simulink model "model_1"  (R2018a)
settings: Solver=VariableStepAuto  StartTime=0.0  StopTime=11  RelTol=1e-3
values from neighbouring files (symbols this model uses):
  Af = 1.8    [script.m]
  Cd = 0.25    [script.m]
  fr = 0.015    [script.m]
  g = 9.81    [script.m]
  Mv = 1310    [script.m]
  rho = 1.2    [script.m]
libraries: simulink x2
settings Model: Creator=Saurabh Suman  LastModifiedBy=Saurabh Suman

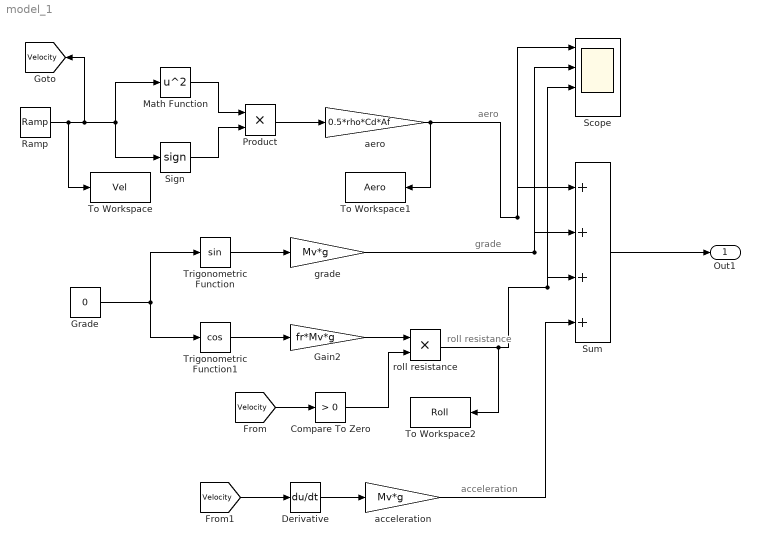
== system model_1 ==
  note: acceleration
  note: roll resistance
  note: grade
  note: aero
  Compare To Zero : simulink/Logic and Bit Operations/Compare To Zero  relop=>  OutDataTypeStr=boolean
  Derivative : Derivative
  Gain2 : Gain  Gain=fr*Mv*g
  Grade : Constant  Value=0
  Math Function : Math  Operator=square  SaturateOnIntegerOverflow=on
  Product : Product
  Ramp : simulink/Sources/Ramp  slope=10  start=1  InitialOutput=0
  Scope : Scope  NumInputPorts=4
  Sign : Signum
  Sum : Sum  Inputs=|++++
  To Workspace : ToWorkspace  VariableName=Vel  SampleTime=-1
      settings: Save2DSignal=2-D array (concatenate along first dimension)
  To Workspace1 : ToWorkspace  VariableName=Aero  SampleTime=-1
      settings: Save2DSignal=2-D array (concatenate along first dimension)
  To Workspace2 : ToWorkspace  VariableName=Roll  SampleTime=-1
      settings: Save2DSignal=2-D array (concatenate along first dimension)
  Trigonometric Function : Trigonometry
  Trigonometric Function1 : Trigonometry  Operator=cos
  acceleration : Gain  Gain=Mv*g
  aero : Gain  Gain=0.5*rho*Cd*Af
  grade : Gain  Gain=Mv*g
  roll resistance : Product
  Out1 : Outport
  tag scope: Velocity=global
  wires:
  Ramp/1 -> To Workspace/1, [Velocity], Sign/1, Math Function/1
  Math Function/1 -> Product/1
  Sign/1 -> Product/2
  Product/1 -> aero/1
  Trigonometric Function1/1 -> Gain2/1
  Trigonometric Function/1 -> grade/1
  Grade/1 -> Trigonometric Function1/1, Trigonometric Function/1
  Gain2/1 -> roll resistance/1
  Compare To Zero/1 -> roll resistance/2
  [Velocity] -> Compare To Zero/1
  aero/1 -> To Workspace1/1, Scope/1, Sum/1
  grade/1 -> Scope/2, Sum/2
  Sum/1 -> Out1/1
  [Velocity] -> Derivative/1
  Derivative/1 -> acceleration/1
  acceleration/1 -> Sum/4
  roll resistance/1 -> To Workspace2/1, Scope/3, Sum/3
